simulink model "AMR_Testing"  (R2023b)
settings: Solver=FixedStepAuto  StartTime=0.0  StopTime=inf  FixedStep=1e-3  RelTol=1e-3
model workspace (MAT data in the model file):
  mdlWSDbList : string (value not decoded)
  min_motor_rpm = 30
  vehicle_track = 877
  vehicle_wheelbase = 2367
  wheel_diameter = 360
  wheel_radius = 180
undefined symbols (not defined in the file or in its folder): Down, Pull
libraries: speedgoatlib_IO60X_IO69X x12, tramontina_database_curtislib x11, tramontina_database_nvidialib x5, simulink x4, tramontina_database_xsenslib x3, speedgoatlib_IO691 x2, simulink_extras x1, tramontina_database_sick_modbuslib x1, canmsglib x1
(part 2 of 2)

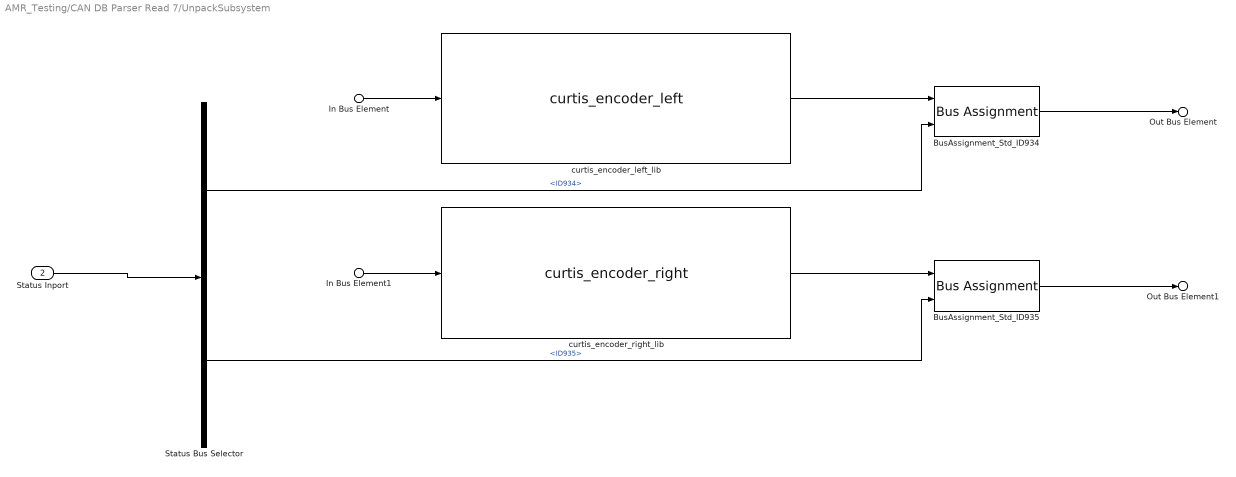
== system AMR_Testing/CAN DB Parser Read 7/UnpackSubsystem ==
  In Bus Element : Inport  PortName=Unpack_In  Element=Std.ID934
  In Bus Element1 : Inport  PortName=Unpack_In  Element=Std.ID935
  Status Inport : Inport  Port=2
  BusAssignment_Std_ID934 : BusAssignment  AssignedSignals=MessageStatus.Status
  BusAssignment_Std_ID935 : BusAssignment  AssignedSignals=MessageStatus.Status
  Status Bus Selector : BusSelector  OutputSignals=Std.ID934,Std.ID935
  curtis_encoder_left_lib : tramontina_database_curtislib/CAN unpack/curtis_encoder_left  SystemSampleTime=-1  VariantActivationTime=update diagram  AllowFlexibleInterface=on  Latency=0  AutoFrameSizeCalculation=off
  curtis_encoder_right_lib : tramontina_database_curtislib/CAN unpack/curtis_encoder_right  SystemSampleTime=-1  VariantActivationTime=update diagram  AllowFlexibleInterface=on  Latency=0  AutoFrameSizeCalculation=off
  Out Bus Element : Outport  PortName=Unpack_Out  Element=ID934_curtis_encoder_left
  Out Bus Element1 : Outport  PortName=Unpack_Out  Element=ID935_curtis_encoder_right
  wires:
  Status Bus Selector/2 -> BusAssignment_Std_ID935/2  "<ID935>"
  Status Bus Selector/1 -> BusAssignment_Std_ID934/2  "<ID934>"
  Status Inport/1 -> Status Bus Selector/1
  BusAssignment_Std_ID935/1 -> Out Bus Element1/1
  curtis_encoder_right_lib/1 -> BusAssignment_Std_ID935/1
  In Bus Element1/1 -> curtis_encoder_right_lib/1
  BusAssignment_Std_ID934/1 -> Out Bus Element/1
  curtis_encoder_left_lib/1 -> BusAssignment_Std_ID934/1
  In Bus Element/1 -> curtis_encoder_left_lib/1

== system AMR_Testing/CAN DB Parser Read 8/ReadSubsystem ==
  CANRead_Std : speedgoatlib_IO60X_IO69X/CAN/CAN Read   moduleType=IO691  id=1  channel=1  canType=CAN (HS)  messageType=CAN (HS)  useBusOut=on  HasMulRead=Specify by IDs  MsgIDlist=[343]  isEFF=off  LabelInHex=off  enableInput=off  initValues=[691 1 0.05 0 1 1 0 1 2 0 1 343]  ts=50e-3
  Data Type ConversionStd : DataTypeConversion  OutDataTypeStr=uint8  SaturateOnIntegerOverflow=off  RndMeth=Floor
  StdSelector_ : Selector  IndexOptions=Index vector (dialog)  Indices=1  OutputSizes=1
  Std_ : Outport  PortName=Raw_Rx  Element=Std.ID343
  StdStatus_ : Outport  Port=2  PortName=Status_Rx  Element=Std.ID343
  wires:
  CANRead_Std/1 -> Data Type ConversionStd/1
  CANRead_Std/2 -> Std_/1
  Data Type ConversionStd/1 -> StdSelector_/1
  StdSelector_/1 -> StdStatus_/1

== system AMR_Testing/CAN DB Parser Read 8/UnpackSubsystem ==
  In Bus Element : Inport  PortName=Unpack_In  Element=Std.ID343
  Status Inport : Inport  Port=2
  AMR_OperationMode_lib : tramontina_database_nvidialib/CAN unpack/AMR_OperationMode  SystemSampleTime=-1  VariantActivationTime=update diagram  AllowFlexibleInterface=on  Latency=0  AutoFrameSizeCalculation=off
  BusAssignment_Std_ID343 : BusAssignment  AssignedSignals=MessageStatus.Status
  Status Bus Selector : BusSelector  OutputSignals=Std.ID343
  Out Bus Element : Outport  PortName=Unpack_Out  Element=ID343_AMR_OperationMode
  wires:
  In Bus Element/1 -> AMR_OperationMode_lib/1
  AMR_OperationMode_lib/1 -> BusAssignment_Std_ID343/1
  BusAssignment_Std_ID343/1 -> Out Bus Element/1
  Status Inport/1 -> Status Bus Selector/1
  Status Bus Selector/1 -> BusAssignment_Std_ID343/2  "<ID343>"

== system AMR_Testing/CAN DB Parser Read 9/ReadSubsystem ==
  CANRead_Std : speedgoatlib_IO60X_IO69X/CAN/CAN Read   moduleType=IO691  id=1  channel=1  canType=CAN (HS)  messageType=CAN (HS)  useBusOut=on  HasMulRead=Specify by IDs  MsgIDlist=[288]  isEFF=off  LabelInHex=off  enableInput=off  initValues=[691 1 0.005 0 1 1 0 1 2 0 1 288]  ts=5e-3
  Data Type ConversionStd : DataTypeConversion  OutDataTypeStr=uint8  SaturateOnIntegerOverflow=off  RndMeth=Floor
  StdSelector_ : Selector  IndexOptions=Index vector (dialog)  Indices=1  OutputSizes=1
  Std_ : Outport  PortName=Raw_Rx  Element=Std.ID288
  StdStatus_ : Outport  Port=2  PortName=Status_Rx  Element=Std.ID288
  wires:
  CANRead_Std/1 -> Data Type ConversionStd/1
  CANRead_Std/2 -> Std_/1
  Data Type ConversionStd/1 -> StdSelector_/1
  StdSelector_/1 -> StdStatus_/1

== system AMR_Testing/CAN DB Parser Read 9/UnpackSubsystem ==
  In Bus Element : Inport  PortName=Unpack_In  Element=Std.ID288
  Status Inport : Inport  Port=2
  BusAssignment_Std_ID288 : BusAssignment  AssignedSignals=MessageStatus.Status
  Status Bus Selector : BusSelector  OutputSignals=Std.ID288
  mobotic_feedback_pos_lib : tramontina_database_nvidialib/CAN unpack/mobotic_feedback_pos  SystemSampleTime=-1  VariantActivationTime=update diagram  AllowFlexibleInterface=on  Latency=0  AutoFrameSizeCalculation=off
  Out Bus Element : Outport  PortName=Unpack_Out  Element=ID288_mobotic_feedback_pos
  wires:
  In Bus Element/1 -> mobotic_feedback_pos_lib/1
  mobotic_feedback_pos_lib/1 -> BusAssignment_Std_ID288/1
  BusAssignment_Std_ID288/1 -> Out Bus Element/1
  Status Inport/1 -> Status Bus Selector/1
  Status Bus Selector/1 -> BusAssignment_Std_ID288/2  "<ID288>"

== system AMR_Testing/CAN DB Parser Write /BusMapping ==
  signal1 : Inport  PortName=InBus  Element=signal1
  signal2 : Inport  PortName=InBus  Element=signal2
  ID550_curtis_input_message_left.rpm_set_left : Outport  PortName=OutBus  Element=ID550_curtis_input_message_left.rpm_set_left
  ID551_curtis_input_message_right.rpm_set_right : Outport  PortName=OutBus  Element=ID551_curtis_input_message_right.rpm_set_right
  wires:
  signal1/1 -> ID550_curtis_input_message_left.rpm_set_left/1
  signal2/1 -> ID551_curtis_input_message_right.rpm_set_right/1

== system AMR_Testing/CAN DB Parser Write /Convert2BusArray ==
  In1 : Inport  PortName=InBus  Element=ID550_curtis_input_message_left
  In2 : Inport  PortName=InBus  Element=ID551_curtis_input_message_right
  BusArray : Concatenate
  BusArrayOut : Outport
  wires:
  In1/1 -> BusArray/1
  In2/1 -> BusArray/2
  BusArray/1 -> BusArrayOut/1

== system AMR_Testing/CAN DB Parser Write /PackSubsystem ==
  In Bus Element : Inport  PortName=PackIn  Element=ID550_curtis_input_message_left
  In Bus Element2 : Inport  PortName=PackIn  Element=ID551_curtis_input_message_right
  curtis_input_message_left_lib : tramontina_database_curtislib/CAN pack/curtis_input_message_left  SystemSampleTime=-1  VariantActivationTime=update diagram  AllowFlexibleInterface=on  Latency=0  AutoFrameSizeCalculation=off
  curtis_input_message_right_lib : tramontina_database_curtislib/CAN pack/curtis_input_message_right  SystemSampleTime=-1  VariantActivationTime=update diagram  AllowFlexibleInterface=on  Latency=0  AutoFrameSizeCalculation=off
  In Bus Element1 : Outport  PortName=PackOut  Element=ID550_curtis_input_message_left
  In Bus Element3 : Outport  PortName=PackOut  Element=ID551_curtis_input_message_right
  wires:
  In Bus Element/1 -> curtis_input_message_left_lib/1
  curtis_input_message_left_lib/1 -> In Bus Element1/1
  In Bus Element2/1 -> curtis_input_message_right_lib/1
  curtis_input_message_right_lib/1 -> In Bus Element3/1

== system AMR_Testing/CAN DB Parser Write 1/Convert2BusArray ==
  In1 : Inport  PortName=InBus  Element=ID0_curtis_input_operational
  BusArray : Concatenate  NumInputs=1
  BusArrayOut : Outport
  wires:
  In1/1 -> BusArray/1
  BusArray/1 -> BusArrayOut/1

== system AMR_Testing/CAN DB Parser Write 1/InputSubsystem ==
  In1_1 : Inport
  ID0_curtis_input_operational.pre_operational : Outport  PortName=OutBus  Element=ID0_curtis_input_operational.pre_operational
  wires:
  In1_1/1 -> ID0_curtis_input_operational.pre_operational/1

== system AMR_Testing/CAN DB Parser Write 1/PackSubsystem ==
  In Bus Element : Inport  PortName=PackIn  Element=ID0_curtis_input_operational
  curtis_input_operational_lib : tramontina_database_curtislib/CAN pack/curtis_input_operational  SystemSampleTime=-1  VariantActivationTime=update diagram  AllowFlexibleInterface=on  Latency=0  AutoFrameSizeCalculation=off
  In Bus Element1 : Outport  PortName=PackOut  Element=ID0_curtis_input_operational
  wires:
  In Bus Element/1 -> curtis_input_operational_lib/1
  curtis_input_operational_lib/1 -> In Bus Element1/1

== system AMR_Testing/CAN DB Parser Write 2/BusMapping ==
  signal3 : Inport  PortName=InBus  Element=signal3
  signal1 : Inport  PortName=InBus  Element=signal1
  signal2 : Inport  PortName=InBus  Element=signal2
  ID344_OperationMode_feedback.OperationMode_auto : Outport  PortName=OutBus  Element=ID344_OperationMode_feedback.OperationMode_auto
  ID344_OperationMode_feedback.OperationMode_idle : Outport  PortName=OutBus  Element=ID344_OperationMode_feedback.OperationMode_idle
  ID344_OperationMode_feedback.OperationMode_manual : Outport  PortName=OutBus  Element=ID344_OperationMode_feedback.OperationMode_manual
  wires:
  signal3/1 -> ID344_OperationMode_feedback.OperationMode_auto/1
  signal1/1 -> ID344_OperationMode_feedback.OperationMode_idle/1
  signal2/1 -> ID344_OperationMode_feedback.OperationMode_manual/1

== system AMR_Testing/CAN DB Parser Write 2/Convert2BusArray ==
  In1 : Inport  PortName=InBus  Element=ID344_OperationMode_feedback
  BusArray : Concatenate  NumInputs=1
  BusArrayOut : Outport
  wires:
  In1/1 -> BusArray/1
  BusArray/1 -> BusArrayOut/1

== system AMR_Testing/CAN DB Parser Write 2/PackSubsystem ==
  In Bus Element : Inport  PortName=PackIn  Element=ID344_OperationMode_feedback
  OperationMode_feedback_lib : tramontina_database_sick_modbuslib/CAN pack/OperationMode_feedback  SystemSampleTime=-1  VariantActivationTime=update diagram  AllowFlexibleInterface=on  Latency=0  AutoFrameSizeCalculation=off
  In Bus Element1 : Outport  PortName=PackOut  Element=ID344_OperationMode_feedback
  wires:
  In Bus Element/1 -> OperationMode_feedback_lib/1
  OperationMode_feedback_lib/1 -> In Bus Element1/1

== system AMR_Testing/CAN DB Parser Write 3/Convert2BusArray ==
  In1 : Inport  PortName=InBus  Element=ID290_AMR_vehicle_speed
  BusArray : Concatenate  NumInputs=1
  BusArrayOut : Outport
  wires:
  In1/1 -> BusArray/1
  BusArray/1 -> BusArrayOut/1

== system AMR_Testing/CAN DB Parser Write 3/InputSubsystem ==
  In1_1 : Inport
  In1_2 : Inport  Port=2
  ID290_AMR_vehicle_speed.speed_m_per_min : Outport  PortName=OutBus  Element=ID290_AMR_vehicle_speed.speed_m_per_min
  ID290_AMR_vehicle_speed.speed_m_per_s : Outport  PortName=OutBus  Element=ID290_AMR_vehicle_speed.speed_m_per_s
  wires:
  In1_1/1 -> ID290_AMR_vehicle_speed.speed_m_per_min/1
  In1_2/1 -> ID290_AMR_vehicle_speed.speed_m_per_s/1

== system AMR_Testing/CAN DB Parser Write 3/PackSubsystem ==
  In Bus Element : Inport  PortName=PackIn  Element=ID290_AMR_vehicle_speed
  AMR_vehicle_speed_lib : tramontina_database_nvidialib/CAN pack/AMR_vehicle_speed  SystemSampleTime=-1  VariantActivationTime=update diagram  AllowFlexibleInterface=on  Latency=0  AutoFrameSizeCalculation=off
  In Bus Element1 : Outport  PortName=PackOut  Element=ID290_AMR_vehicle_speed
  wires:
  In Bus Element/1 -> AMR_vehicle_speed_lib/1
  AMR_vehicle_speed_lib/1 -> In Bus Element1/1

== matlab function AMR_Testing/MATLAB Function1 ==
  data: Actual_Curve_Angle_Front input; Vehicle_Speed output; RPM_Speed_Left input; RPM_Speed_Right input
function Vehicle_Speed = calculateThrottleSpeed(Actual_Curve_Angle_Front, RPM_Speed_Left, RPM_Speed_Right)

    PAR_Wheel_Base = 877;
    PAR_Drive_Wheel_Offset = PAR_Wheel_Base/2;

    if Actual_Curve_Angle_Front == 0
        Vehicle_Speed = (RPM_Speed_Left + RPM_Speed_Right) / 2;
    elseif Actual_Curve_Angle_Front < 0
        Radius_C = PAR_Wheel_Base / tan(deg2rad(abs(Actual_Curve_Angle_Front)));
        Vehicle_Speed = (RPM_Speed_Left * Radius_C + RPM_Speed_Right * (Radius_C - PAR_Drive_Wheel_Offset)) / (2 * Radius_C - PAR_Drive_Wheel_Offset);
    else
        Radius_C = PAR_Wheel_Base / tan(deg2rad(abs(Actual_Curve_Angle_Front)));
        Vehicle_Speed = (RPM_Speed_Left * Radius_C + RPM_Speed_Right * (Radius_C + PAR_Drive_Wheel_Offset)) / (2 * Radius_C + PAR_Drive_Wheel_Offset);
    end
end

== matlab function AMR_Testing/MATLAB Function ==
  data: Actual_Curve_Angle_Front input; vehicle_speed output; Total_Displacement_Left input; Total_Displacement_Right input
% function vehicle_speed = calculateThrottleSpeed(Actual_Curve_Angle_Front, Total_Displacement_Left, Total_Displacement_Right)
% 
%     PAR_Maximal_Wheel_Speed = 1; % Assuming a default value for PAR_Maximal_Wheel_Speed
%     PAR_Wheel_Base = 877;
% 
%     if Actual_Curve_Angle_Front == 0
%         vehicle_speed = PAR_Maximal_Wheel_Speed;
%     else
%         Radius_Avg = PAR_Wheel_Base / (2 * tan(deg2rad(abs(Actual_Curve_Angle_Front))));
%         vehicle_speed = (PAR_Maximal_Wheel_Speed * Radius_Avg) / (Total_Displacement_Left + Total_Displacement_Right);
%     end
% 
% end
% 
function vehicle_speed = calculateThrottleSpeed(Actual_Curve_Angle_Front, Total_Displacement_Left, Total_Displacement_Right)

    persistent prev_Displacement_Left prev_Displacement_Right
    if isempty(prev_Displacement_Left)
        prev_Displacement_Left = 0;
        prev_Displacement_Right = 0;
    end

    PAR_Maximal_Wheel_Speed = 1; % Assuming a default value for PAR_Maximal_Wheel_Speed
    PAR_Wheel_Base = 877;
    
    if Actual_Curve_Angle_Front == 0
        vehicle_speed = PAR_Maximal_Wheel_Speed;
    else
        Radius_Avg = PAR_Wheel_Base / (2 * tan(deg2rad(abs(Actual_Curve_Angle_Front))));
        delta_Left = Total_Displacement_Left - prev_Displacement_Left;
        delta_Right = Total_Displacement_Right - prev_Displacement_Right;
        if delta_Left == 0 && delta_Right == 0
            vehicle_speed = 0;
        else
            vehicle_speed = (PAR_Maximal_Wheel_Speed * Radius_Avg) / (delta_Left + delta_Right);
        end
    end

    % Update previous displacements
    prev_Displacement_Left = Total_Displacement_Left;
    prev_Displacement_Right = Total_Displacement_Right;

end

== stateflow chart AMR_Testing/AMR_oper_mode_chart ==
  state idle
    entry:
    AMR_idle_mode = 1;
    AMR_manual_mode = 0;
    AMR_auto_mode = 0;
    exit:
    AMR_idle_mode = 0;
  state ManualMode
    entry:
    AMR_idle_mode = 0;
    AMR_manual_mode = 1;
    AMR_auto_mode = 0;
    exit:
    AMR_manual_mode = 0;
  state AutoMode
    entry:
    AMR_idle_mode = 0;
    AMR_manual_mode = 0;
    AMR_auto_mode = 1;
    exit:
    AMR_auto_mode = 0;
  (default) -> idle
  idle -> idle [order 3]
  idle -> (junction 13) [order 2] : [AMR_oper_mode == 4]
  (junction 13) -> AutoMode
  (junction 20) -> idle
  AutoMode -> (junction 20) [order 3]
  ManualMode -> idle [order 3]
  idle -> ManualMode [order 1] : [AMR_oper_mode == 2]
  ManualMode -> ManualMode [order 2] : [AMR_oper_mode == 2]
  AutoMode -> AutoMode [order 1] : [AMR_oper_mode == 4]
  ManualMode -> AutoMode [order 1] : [AMR_oper_mode == 4]
  AutoMode -> ManualMode [order 2] : [AMR_oper_mode == 2]
  data: AMR_idle_mode output; AMR_oper_mode input; AMR_manual_mode output; AMR_auto_mode output
